simulink model "filterN_Delay"  (R2014b)
settings: Solver=ode45  StartTime=0.0  StopTime=15  RelTol=1e-3
undefined symbols (not defined in the file): B, J, k1, k2, k3, Kt, La, Ra
libraries: checkpacklib x1, simulink x1
settings Model: Creator=islam  LastModifiedBy=islam

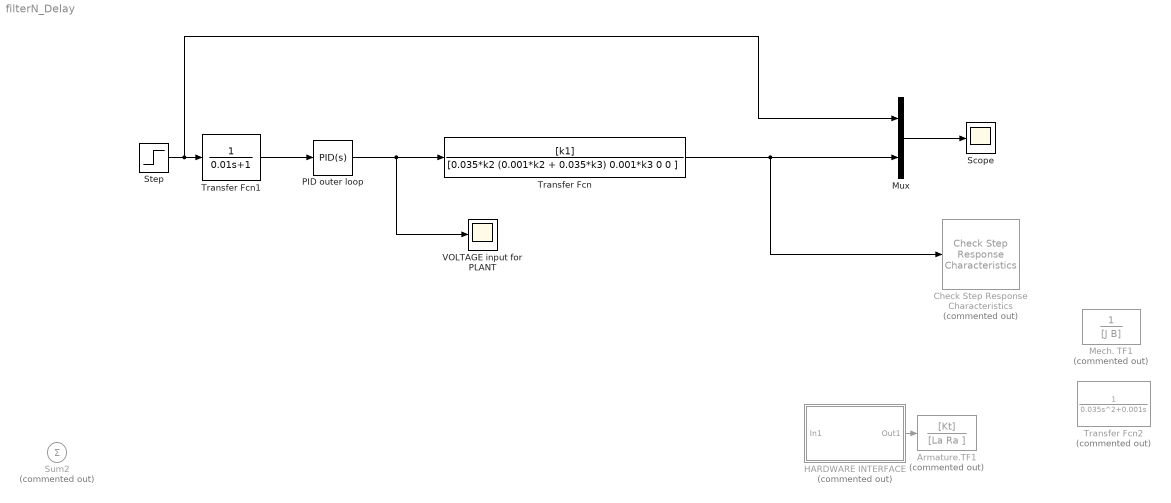
== system filterN_Delay ==
  " VOLTAGE input for PLANT " : Scope
  Armature.TF1 : TransferFcn  Commented=on  Numerator=[Kt]  Denominator=[La Ra ]
  Check Step Response Characteristics : checkpacklib/Check Step Response  Characteristics  Commented=on  InstantiateOnLoad=on  enabled=on  stopWhenAssertionFail=off  export=off  ViewDlgPos=[100 200 510 390]  OpenViewOnLoad=off  LaunchViewOnOpen=on  TimeUnits=seconds  EnableStepResponseBound=on  InitialValue=0  FinalValue=1  StepTime=0  RiseTime=4  PercentRise=80  SettlingTime=6  PercentSettling=1  PercentOvershoot=20  PercentUndershoot=1
  HARDWARE INTERFACE : Subsystem  Commented=on
  Mech. TF1 : TransferFcn  Commented=on  Denominator=[J B]
  Mux : Mux  Inputs=2
  PID outer loop : simulink/Continuous/PID Controller  Controller=PID  TimeDomain=Continuous-time  SampleTime=-1  IntegratorMethod=Forward Euler  FilterMethod=Forward Euler  Form=Parallel  P=1  I=0  D=1  N=0  InitialConditionSource=internal  InitialConditionForIntegrator=0  InitialConditionForFilter=0  ExternalReset=none  LimitOutput=off  UpperSaturationLimit=inf  LowerSaturationLimit=-inf  LinearizeAsGain=on  AntiWindupMode=none  Kb=1  TrackingMode=off  Kt=1  PParamMin=[]  PParamMax=[]  IParamMin=[]  IParamMax=[]  DParamMin=[]  DParamMax=[]  NParamMin=[]  NParamMax=[]  KbParamMin=[]  KbParamMax=[]  KtParamMin=[]  KtParamMax=[]  POutMin=[]  POutMax=[]  IOutMin=[]  IOutMax=[]  DOutMin=[]  DOutMax=[]  NOutMin=[]  NOutMax=[]  KbOutMin=[]  KbOutMax=[]  KtOutMin=[]  KtOutMax=[]  IntegratorOutMin=[]  IntegratorOutMax=[]  FilterOutMin=[]  FilterOutMax=[]  SumOutMin=[]  SumOutMax=[]  SumI1OutMin=[]  SumI1OutMax=[]  SumI2OutMin=[]  SumI2OutMax=[]  SumI3OutMin=[]  SumI3OutMax=[]  SumDOutMin=[]  SumDOutMax=[]  SaturationOutMin=[]  SaturationOutMax=[]  IntegratorContinuousStateAttributes=''  IntegratorStateMustResolveToSignalObject=off  IntegratorRTWStateStorageClass=Auto  FilterContinuousStateAttributes=''  FilterStateMustResolveToSignalObject=off  FilterRTWStateStorageClass=Auto  DifferentiatorICPrevScaledInput=0  DifferentiatorOutMin=[]  DifferentiatorOutMax=[]  UseFilter=on
  Scope : Scope
  Step : Step  SampleTime=0
  Sum2 : Sum  Commented=on  Inputs=|+
  Transfer Fcn : TransferFcn  Numerator=[k1]  Denominator=[0.035*k2 (0.001*k2 + 0.035*k3) 0.001*k3 0 0 ]
  Transfer Fcn1 : TransferFcn  Denominator=[0.01 1]
  Transfer Fcn2 : TransferFcn  Commented=on  Denominator=[0.035 0.001 0]
  wires:
  Step/1 -> Mux/1, Transfer Fcn1/1
  Transfer Fcn1/1 -> PID outer loop/1
  Transfer Fcn/1 -> Mux/2, Check Step Response Characteristics/1
  Mux/1 -> Scope/1
  PID outer loop/1 -> " VOLTAGE input for PLANT "/1, Transfer Fcn/1
  HARDWARE INTERFACE/1(Out1) -> Armature.TF1/1

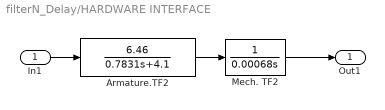
== system filterN_Delay/HARDWARE INTERFACE ==
  In1 : Inport
  Armature.TF2 : TransferFcn  Numerator=[6.46]  Denominator="[0.7831  4.1]"
  Mech. TF2 : TransferFcn  Denominator=[0.00068 0]
  Out1 : Outport
  wires:
  Armature.TF2/1 -> Mech. TF2/1
  In1/1 -> Armature.TF2/1
  Mech. TF2/1 -> Out1/1
